simulink model "mdl_4reac_idealpump_OD"  (R2020b)
settings: Solver=VariableStepAuto  StartTime=0.0  StopTime=stoptime  FixedStep=h  MaxStep=1  RelTol=1e-3  AbsTol=1e-6
undefined symbols (not defined in the file): p
settings Model: Creator=nobel  LastModifiedBy=natha

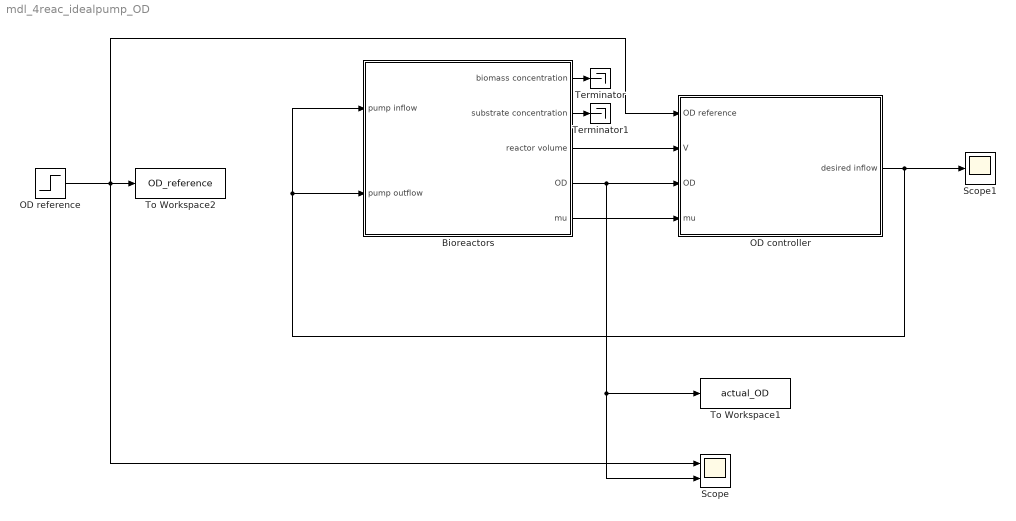
== system mdl_4reac_idealpump_OD ==
  Bioreactors : Subsystem  mask{p=p}
      mask prompts: p "Reactor Parameter Struct"
  OD controller : Subsystem  mask{p=p}
      mask prompts: p "Reactor Parameter Struct"
  OD reference : Step  Time=p.OD.step_time  Before=p.OD.init_val  After=p.OD.final_val  SampleTime=0
  Scope : Scope  NumInputPorts=2
  Scope1 : Scope
  Terminator : Terminator
  Terminator1 : Terminator
  To Workspace1 : ToWorkspace  VariableName=actual_OD  SampleTime=-1
  To Workspace2 : ToWorkspace  VariableName=OD_reference  SampleTime=-1
  wires:
  OD reference/1 -> OD controller/1(OD reference), Scope/1, To Workspace2/1
  Bioreactors/5(mu) -> OD controller/4(mu)
  Bioreactors/4(OD) -> To Workspace1/1, Scope/2, OD controller/3(OD)
  Bioreactors/3(reactor volume) -> OD controller/2(V)
  OD controller/1(desired inflow) -> Scope1/1, Bioreactors/2(pump outflow), Bioreactors/1(pump inflow)
  Bioreactors/1(biomass concentration) -> Terminator/1
  Bioreactors/2(substrate concentration) -> Terminator1/1

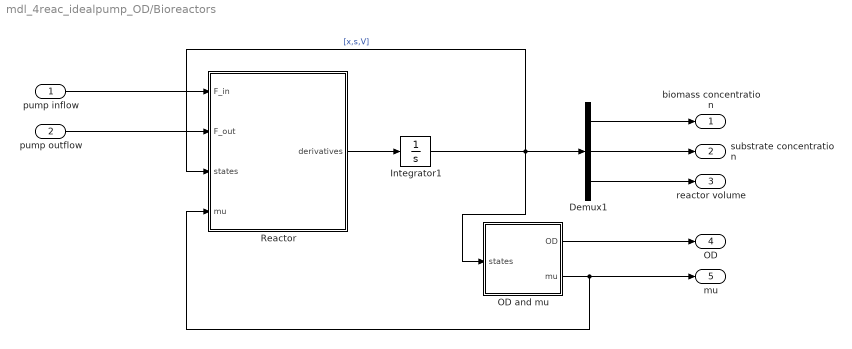
== system mdl_4reac_idealpump_OD/Bioreactors ==
  pump inflow : Inport
  pump outflow : Inport  Port=2
  Demux1 : Demux  Outputs=3
  Integrator1 : Integrator  InitialCondition=[p.init_x; p.init_s; p.init_v];
  OD and mu : MATLAB Function  TreatAsAtomicUnit=on
  Reactor : MATLAB Function  TreatAsAtomicUnit=on
  biomass concentration : Outport
  substrate concentration : Outport  Port=2
  reactor volume : Outport  Port=3
  OD : Outport  Port=4
  mu : Outport  Port=5
  wires:
  pump inflow/1 -> Reactor/1(F_in)
  Demux1/3 -> reactor volume/1
  pump outflow/1 -> Reactor/2(F_out)
  Reactor/1(derivatives) -> Integrator1/1
  OD and mu/2(mu) -> Reactor/4(mu), mu/1
  OD and mu/1(OD) -> OD/1
  Demux1/2 -> substrate concentration/1
  Demux1/1 -> biomass concentration/1
  Integrator1/1 -> Reactor/3(states), Demux1/1, OD and mu/1(states)  "[x,s,V]"

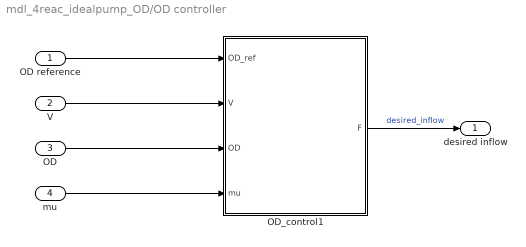
== system mdl_4reac_idealpump_OD/OD controller ==
  OD reference : Inport
  V : Inport  Port=2
  OD : Inport  Port=3
  mu : Inport  Port=4
  OD_control1 : MATLAB Function  TreatAsAtomicUnit=on
  desired inflow : Outport
  wires:
  OD reference/1 -> OD_control1/1(OD_ref)
  mu/1 -> OD_control1/4(mu)
  V/1 -> OD_control1/2(V)
  OD/1 -> OD_control1/3(OD)
  OD_control1/1(F) -> desired inflow/1  "desired_inflow"

== matlab function mdl_4reac_idealpump_OD/OD controller/OD_control1 ==
  data: OD_ref input; V input; F output; OD input; mu input
function F = fcn(OD_ref,V,OD,mu)

F = OD.*mu./OD_ref.*V;

== matlab function mdl_4reac_idealpump_OD/Bioreactors/Reactor ==
  data: F_in input; derivatives output size=3*p.num_reac; F_out input; states input; mu input; p parameter
function derivatives   = fcn(F_in,F_out,states, mu, p)

x=states(1:p.num_reac);
s=states(p.num_reac+(1:p.num_reac));
V=states(2*p.num_reac+(1:p.num_reac));

D = F_in./V;

%dx    (Concentration of biomass in the biorreactor)
dx= mu.*x - D.*x;

%ds    (Concentration of substrate in the biorreactor)
ds= -p.y.*mu.*x + D.*(p.s_f - s);

%dV    (Volume of liquid inside the biorreactor)
dV= F_in - F_out;


derivatives = [dx; ds; dV];

== matlab function mdl_4reac_idealpump_OD/Bioreactors/OD and mu ==
  data: states input; OD output; mu output; p parameter
function [OD,mu] = fcn(states, p)

x=states(1:p.num_reac);
s=states(p.num_reac+(1:p.num_reac));
V=states(2*p.num_reac+(1:p.num_reac));

OD=x./p.m_p./p.nOD;
mu = p.mu_max.*s./(p.K_s+s);
